simulink model "IMC_withboost2007"  (Simulink 7.0)
settings: Solver=ode3  StartTime=0.0  StopTime=Inf  FixedStep=0.1  RelTol=1e-3
settings Model: Creator=ismt  LastModifiedBy=ismt

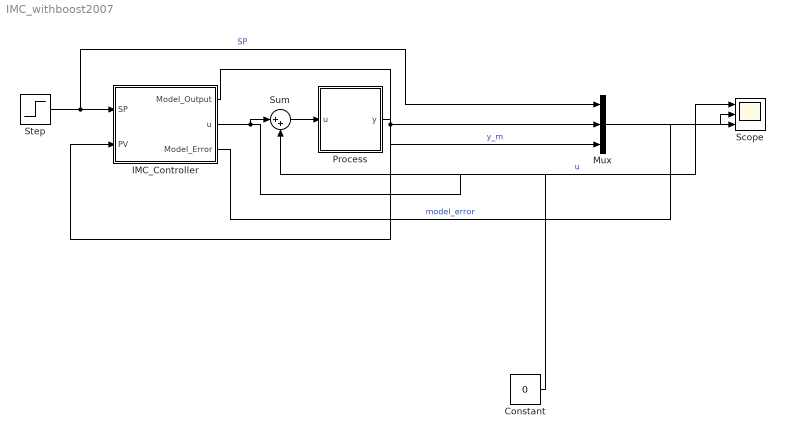
== system IMC_withboost2007 ==
  Constant : Constant  Value=0  OutDataType=sfix(16)  OutScaling=2^0
  IMC_Controller : Subsystem  mask{Kp_hat=1.5, Tau_hat=5, delay_hat=2.5, T_lead=5, T_lag=1}
      mask prompts: Kp_hat "Kp_Model"; Tau_hat "Tau_Model"; delay_hat "Delay_Model"
      mask help:
      | Model Parameters
      | Boost Filter Parameters
  Mux : Mux  Inputs=3
  Process : Subsystem  mask{Kp=2, tau=5, delay=2.5}
      mask help: Process parameters
  Scope : Scope  NumInputPorts=3
      settings: TimeRange=25000  YMin=0~0~0  YMax=19~9.5~2.5
  Step : Step  Time=20  Before=3  After=8  SampleTime=0
  Sum : Sum  Inputs=|++  OutDataType=sfix(16)  OutScaling=2^0
  wires:
  IMC_Controller/2(u) -> Scope/1, Sum/1  "u"
  Process/1(y) -> Mux/2, IMC_Controller/2(PV)
  Step/1 -> IMC_Controller/1(SP), Mux/1  "SP"
  IMC_Controller/1(Model_Output) -> Mux/3  "y_m"
  Mux/1 -> Scope/2
  IMC_Controller/3(Model_Error) -> Scope/3  "model_error"
  Sum/1 -> Process/1(u)
  Constant/1 -> Sum/2

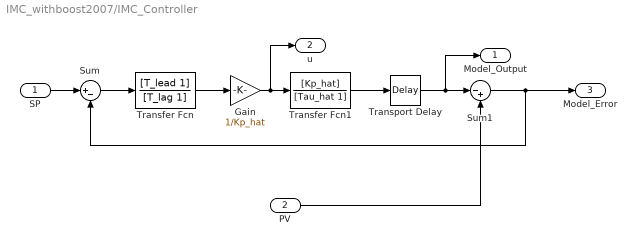
== system IMC_withboost2007/IMC_Controller ==
  SP : Inport  OutDataType=sfix(16)  OutScaling=2^0
  PV : Inport  Port=2  OutDataType=sfix(16)  OutScaling=2^0
  Gain : Gain  Gain=1/Kp_hat  ParameterDataType=sfix(16)  ParameterScaling=2^0  OutDataType=sfix(16)  OutScaling=2^0
  Sum : Sum  Inputs=|+-  OutDataType=sfix(16)  OutScaling=2^0
  Sum1 : Sum  Inputs=|-+  OutDataType=sfix(16)  OutScaling=2^0
  Transfer Fcn : TransferFcn  Numerator=[T_lead 1]  Denominator=[T_lag 1]
  Transfer Fcn1 : TransferFcn  Numerator=[Kp_hat]  Denominator=[Tau_hat 1]
  Transport Delay : TransportDelay  DelayTime=delay_hat
  Model_Output : Outport  OutDataType=sfix(16)  OutScaling=2^0
  u : Outport  Port=2  OutDataType=sfix(16)  OutScaling=2^0
  Model_Error : Outport  Port=3  OutDataType=sfix(16)  OutScaling=2^0
  wires:
  SP/1 -> Sum/1
  Sum/1 -> Transfer Fcn/1
  Transfer Fcn/1 -> Gain/1
  Gain/1 -> Transfer Fcn1/1, u/1
  Transfer Fcn1/1 -> Transport Delay/1
  Transport Delay/1 -> Sum1/1, Model_Output/1
  PV/1 -> Sum1/2
  Sum1/1 -> Model_Error/1, Sum/2

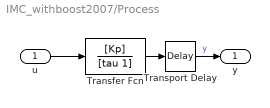
== system IMC_withboost2007/Process ==
  u : Inport
  Transfer Fcn : TransferFcn  Numerator=[Kp]  Denominator=[tau 1]
  Transport Delay : TransportDelay  DelayTime=delay
  y : Outport
  wires:
  Transfer Fcn/1 -> Transport Delay/1
  u/1 -> Transfer Fcn/1
  Transport Delay/1 -> y/1  "y"
